simulink model "joystick"  (Simulink 6.6)
settings: Solver=ode3  StartTime=0.0  StopTime=100000  FixedStep=.01  RelTol=1e-3
libraries: gaugeslibv2 x3, vrlib x1
settings Model: Creator=Administrator  LastModifiedBy=Administrator

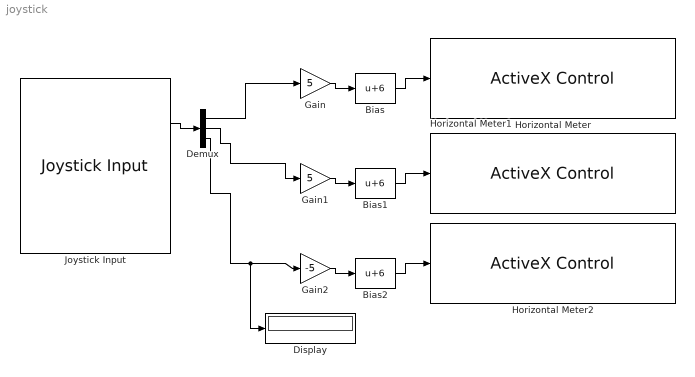
== system joystick ==
  Bias : Bias  Bias=6
  Bias1 : Bias  Bias=6
  Bias2 : Bias  Bias=6
  Demux : Demux  Outputs=3
  Display : Display
  Gain : Gain  Gain=5
  Gain1 : Gain  Gain=5
  Gain2 : Gain  Gain=-5
  Horizontal Meter : gaugeslibv2/ActiveX Control  progid=MWLED.ledctrl.1  connect=input  input=Value  init=hActx.configuration='LED\Sets\Horizontal\Rectangle Horizontal Bitmaps';hActx.Mode=0;hActx.value=0;hActx.Mode=0;hActx.MouseControl=0;  inblock=on  border=on  updateParam=0
  Horizontal Meter1 : gaugeslibv2/ActiveX Control  progid=MWLED.ledctrl.1  connect=input  input=Value  init=hActx.configuration='LED\Sets\Horizontal\Rectangle Horizontal Bitmaps';hActx.Mode=0;hActx.value=0;hActx.Mode=0;hActx.MouseControl=0;  inblock=on  border=on  updateParam=0
  Horizontal Meter2 : gaugeslibv2/ActiveX Control  progid=MWLED.ledctrl.1  connect=input  input=Value  init=hActx.configuration='LED\Sets\Horizontal\Rectangle Horizontal Bitmaps';hActx.Mode=0;hActx.value=0;hActx.Mode=0;hActx.MouseControl=0;  inblock=on  border=on  updateParam=0
  Joystick Input : vrlib/Joystick Input  joyid=0  adjustports=on  forcefeed=off
  wires:
  Joystick Input/1 -> Demux/1
  Demux/2 -> Gain1/1
  Demux/3 -> Gain2/1, Display/1
  Demux/1 -> Gain/1
  Gain/1 -> Bias/1
  Bias/1 -> Horizontal Meter/1
  Gain1/1 -> Bias1/1
  Bias1/1 -> Horizontal Meter1/1
  Gain2/1 -> Bias2/1
  Bias2/1 -> Horizontal Meter2/1
